simulink model "Lab2_2"  (R2022a)
settings: Solver=VariableStepAuto  StartTime=0.0  StopTime=10.0  RelTol=1e-3
settings Model: Creator=Dubov  LastModifiedBy=Dubov

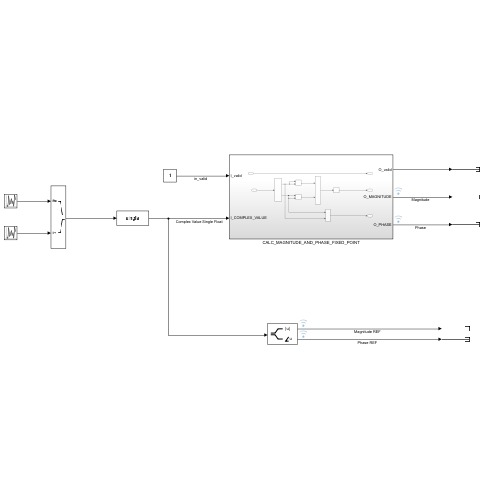
[thumbnail: Simulink's stored preview of the top-level diagram]
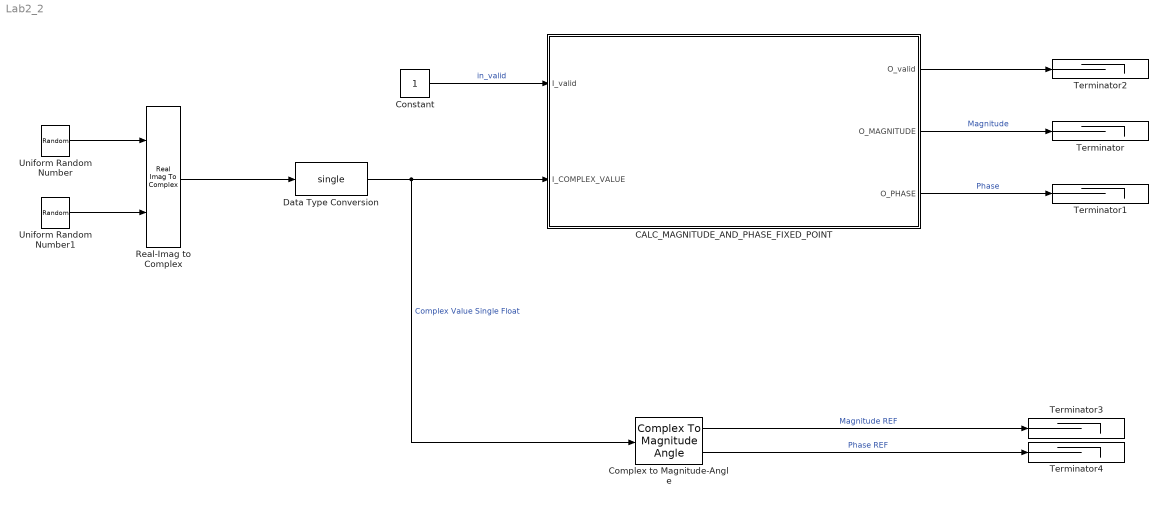
== system Lab2_2 ==
  CALC_MAGNITUDE_AND_PHASE_FIXED_POINT : Subsystem
  Complex to Magnitude-Angle : ComplexToMagnitudeAngle
  Constant : Constant  OutDataTypeStr=boolean
  Data Type Conversion : DataTypeConversion  OutDataTypeStr=single  RndMeth=Round  SaturateOnIntegerOverflow=off
  Real-Imag to Complex : RealImagToComplex
  Terminator{,1..4} (5 alike) : Terminator
  Uniform Random Number : UniformRandomNumber  Minimum=0  Maximum=2^(20)-1  Seed=20  SampleTime=1
  Uniform Random Number1 : UniformRandomNumber  Minimum=0  Maximum=2^(20)-1  Seed=21  SampleTime=1
  wires:
  Constant/1 -> CALC_MAGNITUDE_AND_PHASE_FIXED_POINT/1(I_valid)  "in_valid"
  Data Type Conversion/1 -> CALC_MAGNITUDE_AND_PHASE_FIXED_POINT/2(I_COMPLEX_VALUE), Complex to Magnitude-Angle/1  "Complex Value Single Float"
  CALC_MAGNITUDE_AND_PHASE_FIXED_POINT/3(O_PHASE) -> Terminator1/1  "Phase"
  CALC_MAGNITUDE_AND_PHASE_FIXED_POINT/2(O_MAGNITUDE) -> Terminator/1  "Magnitude"
  CALC_MAGNITUDE_AND_PHASE_FIXED_POINT/1(O_valid) -> Terminator2/1
  Real-Imag to Complex/1 -> Data Type Conversion/1
  Complex to Magnitude-Angle/1 -> Terminator3/1  "Magnitude REF"
  Uniform Random Number1/1 -> Real-Imag to Complex/2
  Uniform Random Number/1 -> Real-Imag to Complex/1
  Complex to Magnitude-Angle/2 -> Terminator4/1  "Phase REF"

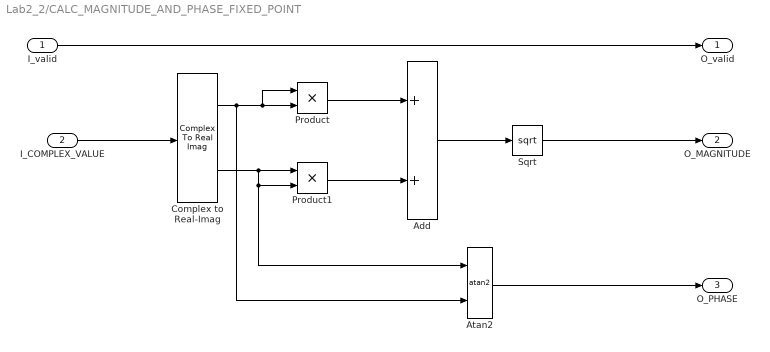
== system Lab2_2/CALC_MAGNITUDE_AND_PHASE_FIXED_POINT ==
  I_valid : Inport
  I_COMPLEX_VALUE : Inport  Port=2
  Add : Sum
  Atan2 : Trigonometry  Operator=atan2  ApproximationMethod=CORDIC
  Complex to Real-Imag : ComplexToRealImag
  Product : Product
  Product1 : Product
  Sqrt : Sqrt  OutDataTypeStr=Inherit: Inherit via internal rule
  O_valid : Outport
  O_MAGNITUDE : Outport  Port=2
  O_PHASE : Outport  Port=3
  wires:
  Complex to Real-Imag/2 -> Atan2/1, Product1/2, Product1/1
  Complex to Real-Imag/1 -> Atan2/2, Product/1, Product/2
  Product1/1 -> Add/2
  Product/1 -> Add/1
  Add/1 -> Sqrt/1
  I_COMPLEX_VALUE/1 -> Complex to Real-Imag/1
  Atan2/1 -> O_PHASE/1
  Sqrt/1 -> O_MAGNITUDE/1
  I_valid/1 -> O_valid/1
